simulink model "minMaxNeuralProcessor"  (R2012b)
settings: Solver=FixedStepDiscrete  StartTime=0.0  StopTime=10.0  RelTol=1e-3
undefined symbols (not defined in the file): dfilt
libraries: dsparch4 x1
settings Model: BufferReuse=off  Creator=gilja  LastModifiedBy=NPTL
settings SolverCC: EnableConcurrentExecution=on  ConcurrentTasks=on
settings DataIOCC: SaveOutput=off  SignalLogging=off  DSMLogging=off  SaveTime=off
settings OptimizationCC: InlineParams=on  InlineInvariantSignals=on  OptimizeBlockIOStorage=off  BufferReuse=off  ExpressionFolding=off  LocalBlockOutputs=off
settings HardwareCC: ProdIntDivRoundTo=Zero  ProdEndianess=LittleEndian  ProdHWDeviceType=Generic->32-bit x86 compatible
settings ModelReferenceCC: ModelReferenceMinAlgLoopOccurrences=on
settings RTWCC: SystemTargetFile=xpctarget.tlc  TemplateMakefile=xpc_default_tmf  Description=xPC Target  ProcessScript=xpctarget_make_rtw_hook  RTWCompilerOptimization=On
settings CodeAppCC: MaxIdLength=62
settings xpcTargetCC: TargetFcnLib=ansi_tfl_table_tmw.mat  CodeReplacementLibrary=XPC_BLAS  ParMdlRefBuildCompliant=on  ConcurrentExecutionCompliant=on  CombineSignalStateStructs=off  GRTInterface=on  xPCTaskExecutionProfile=off  xPCRL32EventNumber=5000  xPCisDownloadable=off  xPCLoadParamSetFile=off  xPCConcurrentTasks=off  xPCEnableSFAnimation=off

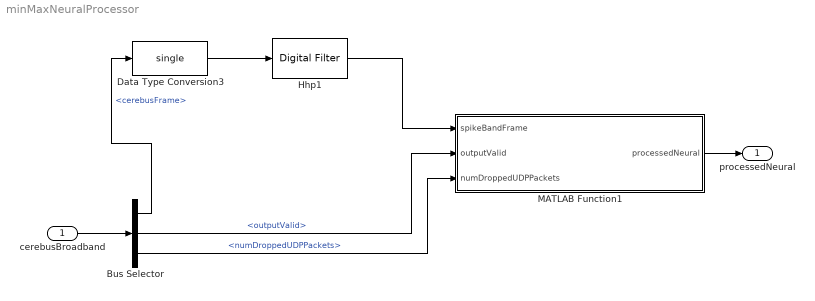
== system minMaxNeuralProcessor ==
  cerebusBroadband : Inport  OutDataTypeStr=Bus: cerebusBroadband
  Bus Selector : BusSelector  OutputSignals=cerebusFrame,outputValid,numDroppedUDPPackets
  Data Type Conversion3 : DataTypeConversion  OutDataTypeStr=single
  Hhp1 : dsparch4/Digital Filter  Tag=BlockMethodSubSystem  TypePopup=FIR (all zeros)  IIRFiltStruct=Direct form II transposed  AllPoleFiltStruct=Direct form  FIRFiltStruct=Direct form  CoeffSource=Specify via dialog  NumCoeffs=[0.086930563487970652 -0.077493493923671095 -0.052086356513811535 -0.036265870077484691 -0.026472273724171571 -0.020391597621137476 -0.016747151929737362 -0.014569789118017987 -0.013306920119703844 -0.012619904125540662 -0.012309352416325515 -0.012205860638726114 -0.012234813425167121 -0.012362066526987289 -0.012579535368795438 -0.012837271062762119 -0.013098379346603142 -0.013340944216534881 -0.013582002513971972 -0.0138223693159251 -0.014064272470618838 -0.014302019489359784 -0.014545406747856631 -0.014779468934346696 -0.014981251463465937 -0.015136716980086347 -0.015281358539846144 -0.015456202829666957 -0.015658337985621749 -0.015831636552543136 -0.015939178736006542 -0.016021502284912441 -0.016138466884829415 -0.016294517404760702 -0.016397223541174257 -0.01643099119707447 -0.016451865300495191 -0.016627358188704266 -0.016658506759097018 -0.016477465876948302 0.98320418059870163 -0.016477465876948302 -0.016658506759097018 -0.016627358188704266 -0.016451865300495191 -0.01643099119707447 -0.016397223541174257 -0.016294517404760702 -0.016138466884829415 -0.016021502284912441 -0.015939178736006542 -0.015831636552543136 -0.015658337985621749 -0.015456202829666957 -0.015281358539846144 -0.015136716980086347 -0.014981251463465937 -0.014779468934346696 -0.014545406747856631 -0.014302019489359784 -0.014064272470618838 -0.0138223693159251 -0.013582002513971972 -0.013340944216534881 -0.013098379346603142 -0.012837271062762119 -0.012579535368795438 -0.012362066526987289 -0.012234813425167121 -0.012205860638726114 -0.012309352416325515 -0.012619904125540662 -0.013306920119703844 -0.014569789118017987 -0.016747151929737362 -0.020391597621137476 -0.026472273724171571 -0.036265870077484691 -0.052086356513811535 -0.077493493923671095 0.086930563487970652]  DenCoeffs=[1 0.1]  BiQuadCoeffs=[1 0.3 0.4 1 0.1 0.2]  LatticeCoeffs=[0.2 0.4]  denIgnore=on  FiltPerSampPopup=One filter per frame  IC=0  ICnum=0  ICden=0  roundingMode=Floor  overflowMode=off  ScaleValues=1  scaleValueFracLength=14  stageInFracLength=15  stageOutFracLength=15  FilterSource=Specify via dialog  dfiltObjectName=dfilt.dffir([1 2 1])  InputProcessing=Columns as channels (frame based)
  MATLAB Function1 : MATLAB Function  TreatAsAtomicUnit=on
  processedNeural : Outport  OutDataTypeStr=Bus: processedNeural  BusOutputAsStruct=on
  wires:
  MATLAB Function1/1(processedNeural) -> processedNeural/1
  cerebusBroadband/1 -> Bus Selector/1
  Bus Selector/1 -> Data Type Conversion3/1  "<cerebusFrame>"
  Bus Selector/2 -> MATLAB Function1/2(outputValid)  "<outputValid>"
  Bus Selector/3 -> MATLAB Function1/3(numDroppedUDPPackets)  "<numDroppedUDPPackets>"
  Hhp1/1 -> MATLAB Function1/1(spikeBandFrame)
  Data Type Conversion3/1 -> Hhp1/1

== matlab function minMaxNeuralProcessor/MATLAB Function1 ==
  data: spikeBandFrame input; outputValid input; numDroppedUDPPackets input; modelConstants parameter; processedNeural output Bus: processedNeural
function processedNeural = extractNerualMaxMin(spikeBandFrame, outputValid, numDroppedUDPPackets, modelConstants)
%#codegen
persistent bufferMeanSquared bufferIdx bufferCnt bufferReady;

if(isempty(bufferCnt))
    bufferCnt = 0;
    bufferIdx = 0;
    bufferMeanSquared = single(zeros(2, size(spikeBandFrame, 2)));
    bufferReady = false;
end

if (bufferCnt == modelConstants.RMSperiod)
    bufferIdx = 1 - bufferIdx;
    bufferMeanSquared(2-bufferIdx, :) = 0;
    bufferCnt = 0;
    bufferReady = true;
end


bufferMeanSquared(2-bufferIdx, :) = bufferMeanSquared(2-bufferIdx, :) + mean(spikeBandFrame.^2) / modelConstants.RMSperiod; 
bufferCnt = bufferCnt + 1;

if(bufferReady && (bufferCnt <= size(spikeBandFrame, 2)))
    processedNeural.meanSquared = bufferMeanSquared(bufferIdx + 1, bufferCnt);
    processedNeural.meanSquaredChannel = uint8(bufferCnt);
else
    processedNeural.meanSquared = single(0);
    processedNeural.meanSquaredChannel = uint8(0);
end
   
   
[processedNeural.minSpikeBand tmpMin] = min(spikeBandFrame);
processedNeural.minSpikeBandInd = uint8(tmpMin);
[processedNeural.maxSpikeBand tmpMax] = max(spikeBandFrame);
processedNeural.maxSpikeBandInd = uint8(tmpMax);
processedNeural.outputValid = outputValid;
processedNeural.numDroppedUDPPackets = numDroppedUDPPackets;
